simulink model "DEF_IEEE14_case2"  (R2022b)
settings: Solver=FixedStepAuto  StartTime=0  StopTime=60  FixedStep=Ts  RelTol=1e-3
StopFcn:
  | data_idq_all_case2 = out.data_idq_all_case2;
  | save('Oscillation_July\data\data_idq_all_case2.mat','data_idq_all_case2');
  | data_vdq_all_case2 = out.data_vdq_all_case2;
  | save('Oscillation_July\data\data_vdq_all_case2.mat','data_vdq_all_case2');
undefined symbols (not defined in the file or in its folder): ApparatusDiscreDamping, ApparatusPara, ApparatusPowerFlow, ApparatusType, Fbase, OtherInputs, Sbase, Ts, Vbase, Wbase, x_e, Ybase, Zbase
libraries: spsGroundLib x22, SimplusGT x22, spsThreePhaseSeriesRLCBranchLib x20, spsThreePhaseParallelRLCBranchLib x14, spsabctoAlphaBetaZeroLib x8, spsThreePhaseTransformerTwoWindingsLib x3, spspowerguiLib x1
(part 2 of 2)

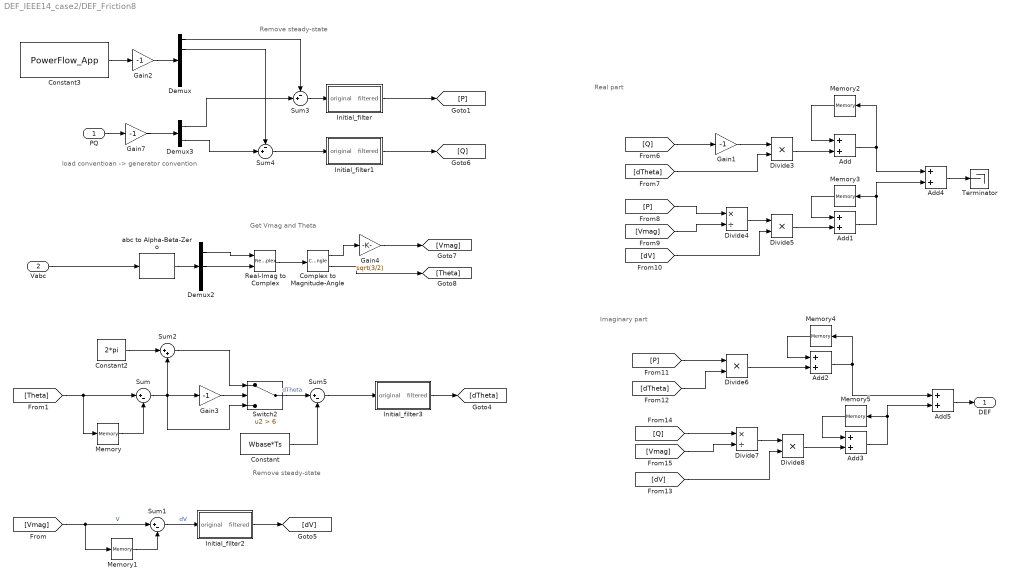
== system DEF_IEEE14_case2/DEF_Friction8 ==
  note: Real part
  note: Imaginary part
  note: load conventioan -> generator convention
  note: Remove steady-state
  note: Remove steady-state
  note: Get Vmag and Theta
  PQ : Inport
  Vabc : Inport  Port=2
  Add{,1..5} (6 alike) : Sum
  Complex to Magnitude-Angle : ComplexToMagnitudeAngle
  Constant : Constant  Value=Wbase*Ts
  Constant2 : Constant  Value=2*pi
  Constant3 : Constant  Value=PowerFlow_App
  Demux : Demux  Outputs=5
  Demux2 : Demux  Outputs=3
  Demux3 : Demux  Outputs=2
  Divide{3,5..6,8} (4 alike) : Product  Inputs=**
  Divide4 : Product  Inputs=*/
  Divide7 : Product  Inputs=*/
  Gain{1..3,7} (4 alike) : Gain  Gain=-1
  Gain4 : Gain  Gain=sqrt(3/2)
  Initial_filter : Subsystem
  Initial_filter1 : Subsystem
  Initial_filter2 : Subsystem
  Initial_filter3 : Subsystem
  Memory{,1..5} (6 alike) : Memory
  Real-Imag to Complex : RealImagToComplex
  Sum : Sum  Inputs=|+-
  Sum1 : Sum  Inputs=|+-
  Sum2 : Sum  Inputs=|++
  Sum3 : Sum  Inputs=-+|
  Sum4 : Sum  Inputs=-+|
  Sum5 : Sum  Inputs=|+-
  Switch2 : Switch  Criteria=u2 > Threshold  Threshold=6  SaturateOnIntegerOverflow=off  InputSameDT=off
  Terminator : Terminator
  abc to Alpha-Beta-Zero : spsabctoAlphaBetaZeroLib/abc to Alpha-Beta-Zero
  DEF : Outport
  wires:
  [Q] -> Divide7/1
  [Vmag] -> Divide4/2
  Divide3/1 -> Add/2
  [P] -> Divide4/1
  [Q] -> Gain1/1
  Gain1/1 -> Divide3/1
  [dTheta] -> Divide3/2
  [dV] -> Divide5/2
  [P] -> Divide6/1
  Divide4/1 -> Divide5/1
  [dTheta] -> Divide6/2
  [dV] -> Divide8/2
  Divide7/1 -> Divide8/1
  [Vmag] -> Divide7/2
  Memory1/1 -> Sum1/2
  [Vmag] -> Memory1/1, Sum1/1  "V"
  Sum1/1 -> Initial_filter2/1(original)  "dV"
  [Theta] -> Sum/1, Memory/1
  Add/1 -> Memory2/1, Add4/1
  Memory2/1 -> Add/1
  Divide5/1 -> Add1/2
  Add1/1 -> Add4/2, Memory3/1
  Memory3/1 -> Add1/1
  Memory4/1 -> Add2/1
  Add2/1 -> Add5/1, Memory4/1
  Divide6/1 -> Add2/2
  Memory5/1 -> Add3/1
  Add3/1 -> Add5/2, Memory5/1
  Divide8/1 -> Add3/2
  Vabc/1 -> abc to Alpha-Beta-Zero/1
  abc to Alpha-Beta-Zero/1 -> Demux2/1
  Memory/1 -> Sum/2
  Sum/1 -> Gain3/1, Switch2/3, Sum2/2
  Sum2/1 -> Switch2/1
  Constant2/1 -> Sum2/1
  Gain3/1 -> Switch2/2
  Constant3/1 -> Gain2/1
  Sum3/1 -> Initial_filter/1(original)
  Demux/1 -> Sum3/1
  Sum4/1 -> Initial_filter1/1(original)
  Demux/2 -> Sum4/1
  Demux3/1 -> Sum3/2
  Demux3/2 -> Sum4/2
  PQ/1 -> Gain7/1
  Initial_filter/1(filtered) -> [P]
  Initial_filter1/1(filtered) -> [Q]
  Initial_filter2/1(filtered) -> [dV]
  Initial_filter3/1(filtered) -> [dTheta]
  Complex to Magnitude-Angle/2 -> [Theta]
  Gain4/1 -> [Vmag]
  Complex to Magnitude-Angle/1 -> Gain4/1
  Real-Imag to Complex/1 -> Complex to Magnitude-Angle/1
  Demux2/1 -> Real-Imag to Complex/1
  Demux2/2 -> Real-Imag to Complex/2
  Gain2/1 -> Demux/1
  Gain7/1 -> Demux3/1
  Switch2/1 -> Sum5/1  "dTheta"
  Sum5/1 -> Initial_filter3/1(original)
  Constant/1 -> Sum5/2
  Add5/1 -> DEF/1
  Add4/1 -> Terminator/1

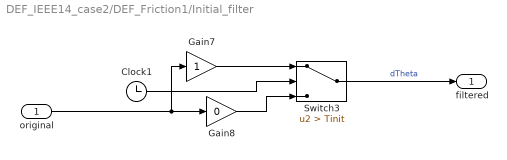
== system DEF_IEEE14_case2/DEF_Friction1/Initial_filter ==
  original : Inport
  Clock1 : Clock
  Gain7 : Gain
  Gain8 : Gain  Gain=0
  Switch3 : Switch  Criteria=u2 > Threshold  Threshold=Tinit  SaturateOnIntegerOverflow=off  InputSameDT=off
  filtered : Outport
  wires:
  Switch3/1 -> filtered/1  "dTheta"
  original/1 -> Gain8/1, Gain7/1
  Gain7/1 -> Switch3/1
  Gain8/1 -> Switch3/3
  Clock1/1 -> Switch3/2

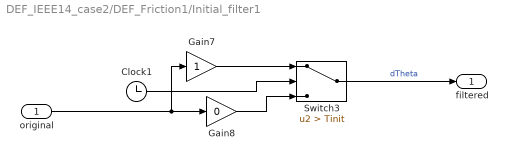
== system DEF_IEEE14_case2/DEF_Friction1/Initial_filter1 ==
  original : Inport
  Clock1 : Clock
  Gain7 : Gain
  Gain8 : Gain  Gain=0
  Switch3 : Switch  Criteria=u2 > Threshold  Threshold=Tinit  SaturateOnIntegerOverflow=off  InputSameDT=off
  filtered : Outport
  wires:
  Switch3/1 -> filtered/1  "dTheta"
  original/1 -> Gain8/1, Gain7/1
  Gain7/1 -> Switch3/1
  Gain8/1 -> Switch3/3
  Clock1/1 -> Switch3/2

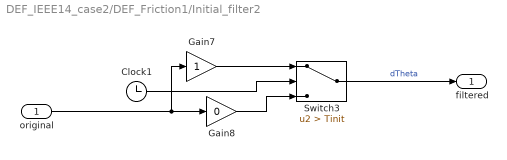
== system DEF_IEEE14_case2/DEF_Friction1/Initial_filter2 ==
  original : Inport
  Clock1 : Clock
  Gain7 : Gain
  Gain8 : Gain  Gain=0
  Switch3 : Switch  Criteria=u2 > Threshold  Threshold=Tinit  SaturateOnIntegerOverflow=off  InputSameDT=off
  filtered : Outport
  wires:
  Switch3/1 -> filtered/1  "dTheta"
  original/1 -> Gain8/1, Gain7/1
  Gain7/1 -> Switch3/1
  Gain8/1 -> Switch3/3
  Clock1/1 -> Switch3/2

== system DEF_IEEE14_case2/DEF_Friction1/Initial_filter3 ==
  original : Inport
  Clock1 : Clock
  Gain7 : Gain
  Gain8 : Gain  Gain=0
  Switch3 : Switch  Criteria=u2 > Threshold  Threshold=Tinit  SaturateOnIntegerOverflow=off  InputSameDT=off
  filtered : Outport
  wires:
  Switch3/1 -> filtered/1  "dTheta"
  original/1 -> Gain8/1, Gain7/1
  Gain7/1 -> Switch3/1
  Gain8/1 -> Switch3/3
  Clock1/1 -> Switch3/2

== system DEF_IEEE14_case2/DEF_Friction2/Initial_filter ==
  original : Inport
  Clock1 : Clock
  Gain7 : Gain
  Gain8 : Gain  Gain=0
  Switch3 : Switch  Criteria=u2 > Threshold  Threshold=Tinit  SaturateOnIntegerOverflow=off  InputSameDT=off
  filtered : Outport
  wires:
  Switch3/1 -> filtered/1  "dTheta"
  original/1 -> Gain8/1, Gain7/1
  Gain7/1 -> Switch3/1
  Gain8/1 -> Switch3/3
  Clock1/1 -> Switch3/2

== system DEF_IEEE14_case2/DEF_Friction2/Initial_filter1 ==
  original : Inport
  Clock1 : Clock
  Gain7 : Gain
  Gain8 : Gain  Gain=0
  Switch3 : Switch  Criteria=u2 > Threshold  Threshold=Tinit  SaturateOnIntegerOverflow=off  InputSameDT=off
  filtered : Outport
  wires:
  Switch3/1 -> filtered/1  "dTheta"
  original/1 -> Gain8/1, Gain7/1
  Gain7/1 -> Switch3/1
  Gain8/1 -> Switch3/3
  Clock1/1 -> Switch3/2

== system DEF_IEEE14_case2/DEF_Friction2/Initial_filter2 ==
  original : Inport
  Clock1 : Clock
  Gain7 : Gain
  Gain8 : Gain  Gain=0
  Switch3 : Switch  Criteria=u2 > Threshold  Threshold=Tinit  SaturateOnIntegerOverflow=off  InputSameDT=off
  filtered : Outport
  wires:
  Switch3/1 -> filtered/1  "dTheta"
  original/1 -> Gain8/1, Gain7/1
  Gain7/1 -> Switch3/1
  Gain8/1 -> Switch3/3
  Clock1/1 -> Switch3/2

== system DEF_IEEE14_case2/DEF_Friction2/Initial_filter3 ==
  original : Inport
  Clock1 : Clock
  Gain7 : Gain
  Gain8 : Gain  Gain=0
  Switch3 : Switch  Criteria=u2 > Threshold  Threshold=Tinit  SaturateOnIntegerOverflow=off  InputSameDT=off
  filtered : Outport
  wires:
  Switch3/1 -> filtered/1  "dTheta"
  original/1 -> Gain8/1, Gain7/1
  Gain7/1 -> Switch3/1
  Gain8/1 -> Switch3/3
  Clock1/1 -> Switch3/2

== system DEF_IEEE14_case2/DEF_Friction3/Initial_filter ==
  original : Inport
  Clock1 : Clock
  Gain7 : Gain
  Gain8 : Gain  Gain=0
  Switch3 : Switch  Criteria=u2 > Threshold  Threshold=Tinit  SaturateOnIntegerOverflow=off  InputSameDT=off
  filtered : Outport
  wires:
  Switch3/1 -> filtered/1  "dTheta"
  original/1 -> Gain8/1, Gain7/1
  Gain7/1 -> Switch3/1
  Gain8/1 -> Switch3/3
  Clock1/1 -> Switch3/2

== system DEF_IEEE14_case2/DEF_Friction3/Initial_filter1 ==
  original : Inport
  Clock1 : Clock
  Gain7 : Gain
  Gain8 : Gain  Gain=0
  Switch3 : Switch  Criteria=u2 > Threshold  Threshold=Tinit  SaturateOnIntegerOverflow=off  InputSameDT=off
  filtered : Outport
  wires:
  Switch3/1 -> filtered/1  "dTheta"
  original/1 -> Gain8/1, Gain7/1
  Gain7/1 -> Switch3/1
  Gain8/1 -> Switch3/3
  Clock1/1 -> Switch3/2

== system DEF_IEEE14_case2/DEF_Friction3/Initial_filter2 ==
  original : Inport
  Clock1 : Clock
  Gain7 : Gain
  Gain8 : Gain  Gain=0
  Switch3 : Switch  Criteria=u2 > Threshold  Threshold=Tinit  SaturateOnIntegerOverflow=off  InputSameDT=off
  filtered : Outport
  wires:
  Switch3/1 -> filtered/1  "dTheta"
  original/1 -> Gain8/1, Gain7/1
  Gain7/1 -> Switch3/1
  Gain8/1 -> Switch3/3
  Clock1/1 -> Switch3/2

== system DEF_IEEE14_case2/DEF_Friction3/Initial_filter3 ==
  original : Inport
  Clock1 : Clock
  Gain7 : Gain
  Gain8 : Gain  Gain=0
  Switch3 : Switch  Criteria=u2 > Threshold  Threshold=Tinit  SaturateOnIntegerOverflow=off  InputSameDT=off
  filtered : Outport
  wires:
  Switch3/1 -> filtered/1  "dTheta"
  original/1 -> Gain8/1, Gain7/1
  Gain7/1 -> Switch3/1
  Gain8/1 -> Switch3/3
  Clock1/1 -> Switch3/2

== system DEF_IEEE14_case2/DEF_Friction4/Initial_filter ==
  original : Inport
  Clock1 : Clock
  Gain7 : Gain
  Gain8 : Gain  Gain=0
  Switch3 : Switch  Criteria=u2 > Threshold  Threshold=Tinit  SaturateOnIntegerOverflow=off  InputSameDT=off
  filtered : Outport
  wires:
  Switch3/1 -> filtered/1  "dTheta"
  original/1 -> Gain8/1, Gain7/1
  Gain7/1 -> Switch3/1
  Gain8/1 -> Switch3/3
  Clock1/1 -> Switch3/2

== system DEF_IEEE14_case2/DEF_Friction4/Initial_filter1 ==
  original : Inport
  Clock1 : Clock
  Gain7 : Gain
  Gain8 : Gain  Gain=0
  Switch3 : Switch  Criteria=u2 > Threshold  Threshold=Tinit  SaturateOnIntegerOverflow=off  InputSameDT=off
  filtered : Outport
  wires:
  Switch3/1 -> filtered/1  "dTheta"
  original/1 -> Gain8/1, Gain7/1
  Gain7/1 -> Switch3/1
  Gain8/1 -> Switch3/3
  Clock1/1 -> Switch3/2

== system DEF_IEEE14_case2/DEF_Friction4/Initial_filter2 ==
  original : Inport
  Clock1 : Clock
  Gain7 : Gain
  Gain8 : Gain  Gain=0
  Switch3 : Switch  Criteria=u2 > Threshold  Threshold=Tinit  SaturateOnIntegerOverflow=off  InputSameDT=off
  filtered : Outport
  wires:
  Switch3/1 -> filtered/1  "dTheta"
  original/1 -> Gain8/1, Gain7/1
  Gain7/1 -> Switch3/1
  Gain8/1 -> Switch3/3
  Clock1/1 -> Switch3/2

== system DEF_IEEE14_case2/DEF_Friction4/Initial_filter3 ==
  original : Inport
  Clock1 : Clock
  Gain7 : Gain
  Gain8 : Gain  Gain=0
  Switch3 : Switch  Criteria=u2 > Threshold  Threshold=Tinit  SaturateOnIntegerOverflow=off  InputSameDT=off
  filtered : Outport
  wires:
  Switch3/1 -> filtered/1  "dTheta"
  original/1 -> Gain8/1, Gain7/1
  Gain7/1 -> Switch3/1
  Gain8/1 -> Switch3/3
  Clock1/1 -> Switch3/2

== system DEF_IEEE14_case2/DEF_Friction5/Initial_filter ==
  original : Inport
  Clock1 : Clock
  Gain7 : Gain
  Gain8 : Gain  Gain=0
  Switch3 : Switch  Criteria=u2 > Threshold  Threshold=Tinit  SaturateOnIntegerOverflow=off  InputSameDT=off
  filtered : Outport
  wires:
  Switch3/1 -> filtered/1  "dTheta"
  original/1 -> Gain8/1, Gain7/1
  Gain7/1 -> Switch3/1
  Gain8/1 -> Switch3/3
  Clock1/1 -> Switch3/2

== system DEF_IEEE14_case2/DEF_Friction5/Initial_filter1 ==
  original : Inport
  Clock1 : Clock
  Gain7 : Gain
  Gain8 : Gain  Gain=0
  Switch3 : Switch  Criteria=u2 > Threshold  Threshold=Tinit  SaturateOnIntegerOverflow=off  InputSameDT=off
  filtered : Outport
  wires:
  Switch3/1 -> filtered/1  "dTheta"
  original/1 -> Gain8/1, Gain7/1
  Gain7/1 -> Switch3/1
  Gain8/1 -> Switch3/3
  Clock1/1 -> Switch3/2

== system DEF_IEEE14_case2/DEF_Friction5/Initial_filter2 ==
  original : Inport
  Clock1 : Clock
  Gain7 : Gain
  Gain8 : Gain  Gain=0
  Switch3 : Switch  Criteria=u2 > Threshold  Threshold=Tinit  SaturateOnIntegerOverflow=off  InputSameDT=off
  filtered : Outport
  wires:
  Switch3/1 -> filtered/1  "dTheta"
  original/1 -> Gain8/1, Gain7/1
  Gain7/1 -> Switch3/1
  Gain8/1 -> Switch3/3
  Clock1/1 -> Switch3/2

== system DEF_IEEE14_case2/DEF_Friction5/Initial_filter3 ==
  original : Inport
  Clock1 : Clock
  Gain7 : Gain
  Gain8 : Gain  Gain=0
  Switch3 : Switch  Criteria=u2 > Threshold  Threshold=Tinit  SaturateOnIntegerOverflow=off  InputSameDT=off
  filtered : Outport
  wires:
  Switch3/1 -> filtered/1  "dTheta"
  original/1 -> Gain8/1, Gain7/1
  Gain7/1 -> Switch3/1
  Gain8/1 -> Switch3/3
  Clock1/1 -> Switch3/2

== system DEF_IEEE14_case2/DEF_Friction6/Initial_filter ==
  original : Inport
  Clock1 : Clock
  Gain7 : Gain
  Gain8 : Gain  Gain=0
  Switch3 : Switch  Criteria=u2 > Threshold  Threshold=Tinit  SaturateOnIntegerOverflow=off  InputSameDT=off
  filtered : Outport
  wires:
  Switch3/1 -> filtered/1  "dTheta"
  original/1 -> Gain8/1, Gain7/1
  Gain7/1 -> Switch3/1
  Gain8/1 -> Switch3/3
  Clock1/1 -> Switch3/2

== system DEF_IEEE14_case2/DEF_Friction6/Initial_filter1 ==
  original : Inport
  Clock1 : Clock
  Gain7 : Gain
  Gain8 : Gain  Gain=0
  Switch3 : Switch  Criteria=u2 > Threshold  Threshold=Tinit  SaturateOnIntegerOverflow=off  InputSameDT=off
  filtered : Outport
  wires:
  Switch3/1 -> filtered/1  "dTheta"
  original/1 -> Gain8/1, Gain7/1
  Gain7/1 -> Switch3/1
  Gain8/1 -> Switch3/3
  Clock1/1 -> Switch3/2

== system DEF_IEEE14_case2/DEF_Friction6/Initial_filter2 ==
  original : Inport
  Clock1 : Clock
  Gain7 : Gain
  Gain8 : Gain  Gain=0
  Switch3 : Switch  Criteria=u2 > Threshold  Threshold=Tinit  SaturateOnIntegerOverflow=off  InputSameDT=off
  filtered : Outport
  wires:
  Switch3/1 -> filtered/1  "dTheta"
  original/1 -> Gain8/1, Gain7/1
  Gain7/1 -> Switch3/1
  Gain8/1 -> Switch3/3
  Clock1/1 -> Switch3/2

== system DEF_IEEE14_case2/DEF_Friction6/Initial_filter3 ==
  original : Inport
  Clock1 : Clock
  Gain7 : Gain
  Gain8 : Gain  Gain=0
  Switch3 : Switch  Criteria=u2 > Threshold  Threshold=Tinit  SaturateOnIntegerOverflow=off  InputSameDT=off
  filtered : Outport
  wires:
  Switch3/1 -> filtered/1  "dTheta"
  original/1 -> Gain8/1, Gain7/1
  Gain7/1 -> Switch3/1
  Gain8/1 -> Switch3/3
  Clock1/1 -> Switch3/2

== system DEF_IEEE14_case2/DEF_Friction7/Initial_filter ==
  original : Inport
  Clock1 : Clock
  Gain7 : Gain
  Gain8 : Gain  Gain=0
  Switch3 : Switch  Criteria=u2 > Threshold  Threshold=Tinit  SaturateOnIntegerOverflow=off  InputSameDT=off
  filtered : Outport
  wires:
  Switch3/1 -> filtered/1  "dTheta"
  original/1 -> Gain8/1, Gain7/1
  Gain7/1 -> Switch3/1
  Gain8/1 -> Switch3/3
  Clock1/1 -> Switch3/2

== system DEF_IEEE14_case2/DEF_Friction7/Initial_filter1 ==
  original : Inport
  Clock1 : Clock
  Gain7 : Gain
  Gain8 : Gain  Gain=0
  Switch3 : Switch  Criteria=u2 > Threshold  Threshold=Tinit  SaturateOnIntegerOverflow=off  InputSameDT=off
  filtered : Outport
  wires:
  Switch3/1 -> filtered/1  "dTheta"
  original/1 -> Gain8/1, Gain7/1
  Gain7/1 -> Switch3/1
  Gain8/1 -> Switch3/3
  Clock1/1 -> Switch3/2

== system DEF_IEEE14_case2/DEF_Friction7/Initial_filter2 ==
  original : Inport
  Clock1 : Clock
  Gain7 : Gain
  Gain8 : Gain  Gain=0
  Switch3 : Switch  Criteria=u2 > Threshold  Threshold=Tinit  SaturateOnIntegerOverflow=off  InputSameDT=off
  filtered : Outport
  wires:
  Switch3/1 -> filtered/1  "dTheta"
  original/1 -> Gain8/1, Gain7/1
  Gain7/1 -> Switch3/1
  Gain8/1 -> Switch3/3
  Clock1/1 -> Switch3/2

== system DEF_IEEE14_case2/DEF_Friction7/Initial_filter3 ==
  original : Inport
  Clock1 : Clock
  Gain7 : Gain
  Gain8 : Gain  Gain=0
  Switch3 : Switch  Criteria=u2 > Threshold  Threshold=Tinit  SaturateOnIntegerOverflow=off  InputSameDT=off
  filtered : Outport
  wires:
  Switch3/1 -> filtered/1  "dTheta"
  original/1 -> Gain8/1, Gain7/1
  Gain7/1 -> Switch3/1
  Gain8/1 -> Switch3/3
  Clock1/1 -> Switch3/2

== system DEF_IEEE14_case2/DEF_Friction8/Initial_filter ==
  original : Inport
  Clock1 : Clock
  Gain7 : Gain
  Gain8 : Gain  Gain=0
  Switch3 : Switch  Criteria=u2 > Threshold  Threshold=Tinit  SaturateOnIntegerOverflow=off  InputSameDT=off
  filtered : Outport
  wires:
  Switch3/1 -> filtered/1  "dTheta"
  original/1 -> Gain8/1, Gain7/1
  Gain7/1 -> Switch3/1
  Gain8/1 -> Switch3/3
  Clock1/1 -> Switch3/2

== system DEF_IEEE14_case2/DEF_Friction8/Initial_filter1 ==
  original : Inport
  Clock1 : Clock
  Gain7 : Gain
  Gain8 : Gain  Gain=0
  Switch3 : Switch  Criteria=u2 > Threshold  Threshold=Tinit  SaturateOnIntegerOverflow=off  InputSameDT=off
  filtered : Outport
  wires:
  Switch3/1 -> filtered/1  "dTheta"
  original/1 -> Gain8/1, Gain7/1
  Gain7/1 -> Switch3/1
  Gain8/1 -> Switch3/3
  Clock1/1 -> Switch3/2

== system DEF_IEEE14_case2/DEF_Friction8/Initial_filter2 ==
  original : Inport
  Clock1 : Clock
  Gain7 : Gain
  Gain8 : Gain  Gain=0
  Switch3 : Switch  Criteria=u2 > Threshold  Threshold=Tinit  SaturateOnIntegerOverflow=off  InputSameDT=off
  filtered : Outport
  wires:
  Switch3/1 -> filtered/1  "dTheta"
  original/1 -> Gain8/1, Gain7/1
  Gain7/1 -> Switch3/1
  Gain8/1 -> Switch3/3
  Clock1/1 -> Switch3/2

== system DEF_IEEE14_case2/DEF_Friction8/Initial_filter3 ==
  original : Inport
  Clock1 : Clock
  Gain7 : Gain
  Gain8 : Gain  Gain=0
  Switch3 : Switch  Criteria=u2 > Threshold  Threshold=Tinit  SaturateOnIntegerOverflow=off  InputSameDT=off
  filtered : Outport
  wires:
  Switch3/1 -> filtered/1  "dTheta"
  original/1 -> Gain8/1, Gain7/1
  Gain7/1 -> Switch3/1
  Gain8/1 -> Switch3/3
  Clock1/1 -> Switch3/2
